simulink model "ppo_position_attitude4drone"  (R2025a)
settings: Solver=ode4  StartTime=0.0  StopTime=50  FixedStep=0.01  RelTol=1e-3
values from neighbouring files (symbols this model uses):
  control_noise = 0.045    [PPO_simulation.mat]    (also in TEST_POS_ATT_PPO.m)
  p_IC = IC(10)    [TEST_POS_ATT_PPO.m]
  phi_IC = IC(7)    [TEST_POS_ATT_PPO.m]
  psi_IC = IC(9)    [TEST_POS_ATT_PPO.m]
  q_IC = IC(11)    [TEST_POS_ATT_PPO.m]
  r_IC = IC(12)    [TEST_POS_ATT_PPO.m]
  state_noise = 0.045    [PPO_simulation.mat]    (also in TEST_POS_ATT_PPO.m)
  theta_IC = IC(8)    [TEST_POS_ATT_PPO.m]
  Ts_Sim = 0.01    [PPO_simulation.mat]    (also in TEST_POS_ATT_PPO.m)
  u_IC = IC(4)    [TEST_POS_ATT_PPO.m]
  v_IC = IC(5)    [TEST_POS_ATT_PPO.m]
  w_IC = IC(6)    [TEST_POS_ATT_PPO.m]
  x_IC = IC(1)    [TEST_POS_ATT_PPO.m]
  y_IC = IC(2)    [TEST_POS_ATT_PPO.m]
  z_IC = IC(3)    [TEST_POS_ATT_PPO.m]
undefined symbols (not defined in the file or in its folder): p_IC2, p_IC3, p_IC4, phi_IC2, phi_IC3, psi_IC2, psi_IC3, q_IC2, q_IC3, r_IC2, r_IC3, saturation_logic, theta_IC2, theta_IC3, u_IC2, u_IC3, v_IC2, v_IC3, w_IC2, w_IC3, wind_logic, x_IC2, x_IC3, y_IC2, y_IC3, z_IC2, z_IC3
libraries: rllib x8
(part 2 of 2)

== matlab function ppo_position_attitude4drone/drone2/Drone_Dynamic1/MATLAB Function5 ==
  data: X input; Wxyz input; X output; Ts_Sim input; wind_logic input
function X = wind_f_m( X,Wxyz, Ts_Sim,  wind_logic)

    Cd = [.8; 0.8;1.2]; % Drag coefficient
    L = 0.2; % Half arm length (m)
    h = 0.05;
    A = [L*2*h, L*2*h, 2*L*L]; % Approximate frontal areas [x, y, z] in m^2
    r = [ L,  L, -L, -L;   % X positions of motors
          L, -L, -L,  L;   % Y positions of motors
          0,  0,  0,  0 ]; % Z positions (motors at same height)
    rho = 1.225; % Air density (kg/m^3)

    Ix = 0.3; Iy = 0.4; Iz = 0.5; m = 1;
    if wind_logic ==1
        R = eul2rotm_zyx( X(7), X(8), X(9) );
        Wxyz_body = R'*Wxyz;
        V_rel = X(4:6) - Wxyz_body;
        F_wind = -0.5 * rho * Cd .*diag(A) * (V_rel .* abs(V_rel)); % Compute wind forces
        
        F_wind_motors = repmat(F_wind, 1, 4) + 0.01*randn(3,4);
    
        M_wind_motors = cross(r, F_wind_motors, 1);
        M_wind = sum(M_wind_motors, 2);  
        
        accn_dist = F_wind/m;
        alpha_dist=    [M_wind(1)/Ix;
                        M_wind(2)/Iy;
                        M_wind(3)/Iz];
    
        X = X + Ts_Sim * [0;0;0;
                         accn_dist;
                         0;0;0;
                         alpha_dist];
    end
end

== matlab function ppo_position_attitude4drone/drone2/Drone_Dynamic1/MATLAB Function6 ==
  data: U input; out output; logic input
% saturation function
function out = saturate_controls(U, logic)

    if logic == 1

        ft = U(1);
        torques = [U(2); U(3); U(4)];
        m = 1;
        g = 9.81;
        L = 0.2;
        drag = 0.02; % (drag coef)
        max_Ft = 2*m*g;
        Tmin = 0;
        Tmax = max_Ft/4;
        max_torque = Tmax*L*2;
        max_yaw_torque = 0.7*max_torque;

        % saturate the torques to the max torque the drone can produce
        for p = 1:2 % sat the first 2
            if torques(p) > max_torque
                torques(p) = max_torque;
            elseif torques(p) < -max_torque
                torques(p) = -max_torque;
            end
        end
        if torques(3) > max_yaw_torque
            torques(3) = max_yaw_torque;
        elseif torques(3) < -max_yaw_torque
            torques(3) = -max_yaw_torque;
        end
        % solve for the thrust of each motor given those torques
        T1 = (ft - torques(1)/(2*L) - torques(2)/(2*L) + torques(3)/(4*drag)) / 4;
        T2 = (ft - torques(1)/(2*L) + torques(2)/(2*L) + torques(3)/(4*drag)) / 4;
        T3 = (ft + torques(1)/(2*L) - torques(2)/(2*L) - torques(3)/(4*drag)) / 4;
        T4 = (ft + torques(1)/(2*L) + torques(2)/(2*L) - torques(3)/(4*drag)) / 4;
        each_motor_thrust = [T1;T2;T3;T4];

        % saturate each motor thrust to its bounded values
        for j = 1:4
            if each_motor_thrust(j) > Tmax
                each_motor_thrust(j) = Tmax;
            elseif each_motor_thrust(j) < Tmin
                each_motor_thrust(j) = Tmin;
            end
        end

        ft = sum(each_motor_thrust);

        if ft>max_Ft
            ft = max_Ft;
        elseif ft<0
            ft = 0;
        end

        out = [ft; torques];

    else
    
        out = U;
    
    end


end

== matlab function ppo_position_attitude4drone/drone2/Drone_Dynamic1/linear transfomation ==
  data: p input; q input; r input; phi_dot output; phi input; theta input; theta_dot output; psi_dot output
function [phi_dot, theta_dot, psi_dot] = fcn(p,q,r, phi,theta)

    phi_dot   = p + (q*sin(phi)*tan(theta)) + (r*cos(phi)*tan(theta));
    theta_dot = (q*cos(phi)) - (r*sin(phi));
    psi_dot   = (q*sin(phi)/cos(theta)) + (r*cos(phi)/cos(theta));

end



    % if theta == deg2rad(90) || theta == deg2rad(-90)
    %    theta = sign(theta)*deg2rad(89.9); 
    % end

% 89.9 value is fixed. 
% if change to 89.99, phi_dot and psi_dot value will explode.

== matlab function ppo_position_attitude4drone/leader drone/PPO_position_controller/Reward Function ==
  data: err input; u input; reward output
function reward  = fcn(err, u)

    % reward = -0.1 * (err.' * Q_pos * err + u.' * R_pos * u);
    err1 = err(1); % x
    err2 = err(2); % x_dot
    err3 = err(3);
    err4 = err(4);
    err5 = err(5);
    err6 = err(6);

    ux = u(1);
    uy = u(2);
    uz = u(3);

    reward = -0.05*(1*abs(err1) + 0.1*abs(err2) + 1*abs(err3) + 0.1*abs(err4) + ...
                    1*abs(err5) + 0.1*abs(err6) + 0.1*abs(ux) + 0.1*abs(uy) + 0.1*abs(uz));

end

== matlab function ppo_position_attitude4drone/drone2/PPO_attitude_controller/MATLAB Function1 ==
  data: err input; reward output; u input
function reward = fcn(err,u)
    err1 = err(1); % phi
    err2 = err(2); % phi_dot
    err3 = err(3);
    err4 = err(4);
    err5 = err(5);
    err6 = err(6);

    ux = u(1);
    uy = u(2);
    uz = u(3);

    reward = -1*(1*abs(err1) + 0.1*abs(err2) + 1*abs(err3) + 0.1*abs(err4) + ...
                    1*abs(err5) + 0.1*abs(err6) + 0.1*abs(ux) + 0.1*abs(uy) + 0.01*abs(uz));

end

== matlab function ppo_position_attitude4drone/drone2/PPO_position_controller/Reward Function ==
  data: err input; u input; reward output
function reward  = fcn(err, u)

    % reward = -0.1 * (err.' * Q_pos * err + u.' * R_pos * u);
    err1 = err(1); % x
    err2 = err(2); % x_dot
    err3 = err(3);
    err4 = err(4);
    err5 = err(5);
    err6 = err(6);

    ux = u(1);
    uy = u(2);
    uz = u(3);

    reward = -0.05*(1*abs(err1) + 0.1*abs(err2) + 1*abs(err3) + 0.1*abs(err4) + ...
                    1*abs(err5) + 0.1*abs(err6) + 0.1*abs(ux) + 0.1*abs(uy) + 0.1*abs(uz));

end

== matlab function ppo_position_attitude4drone/drone2/System_Solver ==
  data: phi_desired output; theta_desired output; psi_desired output; u_x input; Ft_desired output; u_y input; u_z input; t input
function [phi_desired, theta_desired, psi_desired, Ft_desired] = fcn(u_x, u_y, u_z, t)
    
    m = 1;
    psi_desired = 0.09;
    u_z = 9.81-u_z;
    Ft_desired = m * sqrt(u_x^2 + u_y^2 + u_z^2);
    phi_desired = asin((u_y*m)/Ft_desired);
    theta_desired = asin((-u_x*m) / (Ft_desired*cos(phi_desired)));

    %% the method below should work identically, use either 
    % a = sin(psi_desired); %sin(0) = 0
    % b = cos(psi_desired); %cos(0) = 1
    % A = u_x/u_z;
    % B = u_y/u_z;
    % C = (a*A - b*B) / ( (a^2) + (b^2));
    % phi_desired = atan((B + b*C) / a);
    % theta_desired = atan(C * cos(phi_desired));
    %%
    phi_desired = phi_desired *(1-exp(-2*t));
    theta_desired = theta_desired * (1-exp(-2*t));
    if phi_desired > pi/6
        phi_desired = pi/6;
    elseif phi_desired < -pi/6
        phi_desired = -pi/6;
    end
    %%
    if theta_desired > pi/6
        theta_desired = pi/6;
    elseif theta_desired < -pi/6
        theta_desired = -pi/6;
    end
    % Ft_desired = (m / (cos(theta_desired) * cos(phi_desired))) * (-u_z);
end

== matlab function ppo_position_attitude4drone/drone3/Drone_Dynamic1/MATLAB Function ==
  data: tau_x input; tau_y input; tau_z input; phi_d_dot output; theta_d_dot output; psi_d_dot output; phi_dot input; theta_dot input; psi_dot input
function [phi_d_dot, theta_d_dot, psi_d_dot] = fcn(tau_x, tau_y, tau_z, phi_dot, theta_dot, psi_dot)
    I_x = 0.3; I_y = 0.4; I_z = 0.5;
    phi_d_dot = (((I_y - I_z)/I_x) * theta_dot * psi_dot) + (tau_x/I_x);
    theta_d_dot = (((I_z - I_x)/I_y) * phi_dot * psi_dot) + (tau_y/I_y);
    psi_d_dot = (((I_x - I_y)/I_z) * phi_dot * psi_dot) + (tau_z/I_z);
end

== matlab function ppo_position_attitude4drone/drone3/Drone_Dynamic1/MATLAB Function1 ==
  data: phi input; x_d_dot output; theta input; psi input; F_t input; y_d_dot output; z_d_dot output
function [x_d_dot, y_d_dot, z_d_dot] = fcn(phi, theta, psi, F_t)
    m = 1; %1kg
    g = 9.81;
    x_d_dot= -(F_t/m) * (sin(phi)*sin(psi) + cos(phi)*cos(psi)*sin(theta));
    y_d_dot= -(F_t/m) * (cos(phi)*sin(psi)*sin(theta) - cos(psi)*sin(phi));
    z_d_dot= g-(F_t/m) * (cos(phi) * cos(theta));
end

== matlab function ppo_position_attitude4drone/drone3/Drone_Dynamic1/MATLAB Function3 ==
  settings: updateMethod=DISCRETE
  data: state_vector input; noisy_vector output; noise_percent input
function noisy_vector = add_state_noise(state_vector,noise_percent)

    sensor_uncert = [0.02, 0.02, 0.05, 0.05, 0.05, 0.05, 0.15, 0.15, 0.5, 0.005, 0.005, 0.005]';
  
    noise = (noise_percent) * sensor_uncert .* randn(size(state_vector)); % 0.01 usually add noise_percent 1 2 3 4 5
    noisy_vector = state_vector + noise;

end

== matlab function ppo_position_attitude4drone/drone3/Drone_Dynamic1/MATLAB Function4 ==
  settings: updateMethod=DISCRETE
  data: control_vector input; noisy_vector output; noise_percent input
function noisy_vector = add_control_noise(control_vector, noise_percent)

    L = 0.2;
    % drag = 0.02; % (drag coef)
    max_Ft = 2*9.81;
    Tmax = max_Ft/4;
    Max_torque = Tmax*L*2;
    actuator_uncert = [0.1*max_Ft, 0.01*Max_torque, 0.01*Max_torque, 0.02*Max_torque]';
    
    noise = (noise_percent) * actuator_uncert .* randn(size(control_vector)); % noise_percent 1 2 3 4 5
    noisy_vector = control_vector + noise;
    
end

== matlab function ppo_position_attitude4drone/drone3/Drone_Dynamic1/MATLAB Function5 ==
  data: X input; Wxyz input; X output; Ts_Sim input; wind_logic input
function X = wind_f_m( X,Wxyz, Ts_Sim,  wind_logic)

    Cd = [.8; 0.8;1.2]; % Drag coefficient
    L = 0.2; % Half arm length (m)
    h = 0.05;
    A = [L*2*h, L*2*h, 2*L*L]; % Approximate frontal areas [x, y, z] in m^2
    r = [ L,  L, -L, -L;   % X positions of motors
          L, -L, -L,  L;   % Y positions of motors
          0,  0,  0,  0 ]; % Z positions (motors at same height)
    rho = 1.225; % Air density (kg/m^3)

    Ix = 0.3; Iy = 0.4; Iz = 0.5; m = 1;
    if wind_logic ==1
        R = eul2rotm_zyx( X(7), X(8), X(9) );
        Wxyz_body = R'*Wxyz;
        V_rel = X(4:6) - Wxyz_body;
        F_wind = -0.5 * rho * Cd .*diag(A) * (V_rel .* abs(V_rel)); % Compute wind forces
        
        F_wind_motors = repmat(F_wind, 1, 4) + 0.01*randn(3,4);
    
        M_wind_motors = cross(r, F_wind_motors, 1);
        M_wind = sum(M_wind_motors, 2);  
        
        accn_dist = F_wind/m;
        alpha_dist=    [M_wind(1)/Ix;
                        M_wind(2)/Iy;
                        M_wind(3)/Iz];
    
        X = X + Ts_Sim * [0;0;0;
                         accn_dist;
                         0;0;0;
                         alpha_dist];
    end
end

== matlab function ppo_position_attitude4drone/leader drone/System_Solver ==
  data: phi_desired output; theta_desired output; psi_desired output; u_x input; Ft_desired output; u_y input; u_z input; t input
function [phi_desired, theta_desired, psi_desired, Ft_desired] = fcn(u_x, u_y, u_z, t)
    
    m = 1;
    psi_desired = 0.09;
    u_z = 9.81-u_z;
    Ft_desired = m * sqrt(u_x^2 + u_y^2 + u_z^2);
    phi_desired = asin((u_y*m)/Ft_desired);
    theta_desired = asin((-u_x*m) / (Ft_desired*cos(phi_desired)));

    %% the method below should work identically, use either 
    % a = sin(psi_desired); %sin(0) = 0
    % b = cos(psi_desired); %cos(0) = 1
    % A = u_x/u_z;
    % B = u_y/u_z;
    % C = (a*A - b*B) / ( (a^2) + (b^2));
    % phi_desired = atan((B + b*C) / a);
    % theta_desired = atan(C * cos(phi_desired));
    %%
    phi_desired = phi_desired *(1-exp(-2*t));
    theta_desired = theta_desired * (1-exp(-2*t));
    if phi_desired > pi/6
        phi_desired = pi/6;
    elseif phi_desired < -pi/6
        phi_desired = -pi/6;
    end
    %%
    if theta_desired > pi/6
        theta_desired = pi/6;
    elseif theta_desired < -pi/6
        theta_desired = -pi/6;
    end
    % Ft_desired = (m / (cos(theta_desired) * cos(phi_desired))) * (-u_z);
end

== matlab function ppo_position_attitude4drone/drone3/Drone_Dynamic1/MATLAB Function6 ==
  data: U input; out output; logic input
% saturation function
function out = saturate_controls(U, logic)

    if logic == 1

        ft = U(1);
        torques = [U(2); U(3); U(4)];
        m = 1;
        g = 9.81;
        L = 0.2;
        drag = 0.02; % (drag coef)
        max_Ft = 2*m*g;
        Tmin = 0;
        Tmax = max_Ft/4;
        max_torque = Tmax*L*2;
        max_yaw_torque = 0.7*max_torque;

        % saturate the torques to the max torque the drone can produce
        for p = 1:2 % sat the first 2
            if torques(p) > max_torque
                torques(p) = max_torque;
            elseif torques(p) < -max_torque
                torques(p) = -max_torque;
            end
        end
        if torques(3) > max_yaw_torque
            torques(3) = max_yaw_torque;
        elseif torques(3) < -max_yaw_torque
            torques(3) = -max_yaw_torque;
        end
        % solve for the thrust of each motor given those torques
        T1 = (ft - torques(1)/(2*L) - torques(2)/(2*L) + torques(3)/(4*drag)) / 4;
        T2 = (ft - torques(1)/(2*L) + torques(2)/(2*L) + torques(3)/(4*drag)) / 4;
        T3 = (ft + torques(1)/(2*L) - torques(2)/(2*L) - torques(3)/(4*drag)) / 4;
        T4 = (ft + torques(1)/(2*L) + torques(2)/(2*L) - torques(3)/(4*drag)) / 4;
        each_motor_thrust = [T1;T2;T3;T4];

        % saturate each motor thrust to its bounded values
        for j = 1:4
            if each_motor_thrust(j) > Tmax
                each_motor_thrust(j) = Tmax;
            elseif each_motor_thrust(j) < Tmin
                each_motor_thrust(j) = Tmin;
            end
        end

        ft = sum(each_motor_thrust);

        if ft>max_Ft
            ft = max_Ft;
        elseif ft<0
            ft = 0;
        end

        out = [ft; torques];

    else
    
        out = U;
    
    end


end

== matlab function ppo_position_attitude4drone/drone3/Drone_Dynamic1/linear transfomation ==
  data: p input; q input; r input; phi_dot output; phi input; theta input; theta_dot output; psi_dot output
function [phi_dot, theta_dot, psi_dot] = fcn(p,q,r, phi,theta)

    phi_dot   = p + (q*sin(phi)*tan(theta)) + (r*cos(phi)*tan(theta));
    theta_dot = (q*cos(phi)) - (r*sin(phi));
    psi_dot   = (q*sin(phi)/cos(theta)) + (r*cos(phi)/cos(theta));

end



    % if theta == deg2rad(90) || theta == deg2rad(-90)
    %    theta = sign(theta)*deg2rad(89.9); 
    % end

% 89.9 value is fixed. 
% if change to 89.99, phi_dot and psi_dot value will explode.

== matlab function ppo_position_attitude4drone/drone3/PPO_attitude_controller/MATLAB Function1 ==
  data: err input; reward output; u input
function reward = fcn(err,u)
    err1 = err(1); % phi
    err2 = err(2); % phi_dot
    err3 = err(3);
    err4 = err(4);
    err5 = err(5);
    err6 = err(6);

    ux = u(1);
    uy = u(2);
    uz = u(3);

    reward = -1*(1*abs(err1) + 0.1*abs(err2) + 1*abs(err3) + 0.1*abs(err4) + ...
                    1*abs(err5) + 0.1*abs(err6) + 0.1*abs(ux) + 0.1*abs(uy) + 0.01*abs(uz));

end

== matlab function ppo_position_attitude4drone/drone3/PPO_position_controller/Reward Function ==
  data: err input; u input; reward output
function reward  = fcn(err, u)

    % reward = -0.1 * (err.' * Q_pos * err + u.' * R_pos * u);
    err1 = err(1); % x
    err2 = err(2); % x_dot
    err3 = err(3);
    err4 = err(4);
    err5 = err(5);
    err6 = err(6);

    ux = u(1);
    uy = u(2);
    uz = u(3);

    reward = -0.05*(1*abs(err1) + 0.1*abs(err2) + 1*abs(err3) + 0.1*abs(err4) + ...
                    1*abs(err5) + 0.1*abs(err6) + 0.1*abs(ux) + 0.1*abs(uy) + 0.1*abs(uz));

end

== matlab function ppo_position_attitude4drone/drone3/System_Solver ==
  data: phi_desired output; theta_desired output; psi_desired output; u_x input; Ft_desired output; u_y input; u_z input; t input
function [phi_desired, theta_desired, psi_desired, Ft_desired] = fcn(u_x, u_y, u_z, t)
    
    m = 1;
    psi_desired = 0.09;
    u_z = 9.81-u_z;
    Ft_desired = m * sqrt(u_x^2 + u_y^2 + u_z^2);
    phi_desired = asin((u_y*m)/Ft_desired);
    theta_desired = asin((-u_x*m) / (Ft_desired*cos(phi_desired)));

    %% the method below should work identically, use either 
    % a = sin(psi_desired); %sin(0) = 0
    % b = cos(psi_desired); %cos(0) = 1
    % A = u_x/u_z;
    % B = u_y/u_z;
    % C = (a*A - b*B) / ( (a^2) + (b^2));
    % phi_desired = atan((B + b*C) / a);
    % theta_desired = atan(C * cos(phi_desired));
    %%
    phi_desired = phi_desired *(1-exp(-2*t));
    theta_desired = theta_desired * (1-exp(-2*t));
    if phi_desired > pi/6
        phi_desired = pi/6;
    elseif phi_desired < -pi/6
        phi_desired = -pi/6;
    end
    %%
    if theta_desired > pi/6
        theta_desired = pi/6;
    elseif theta_desired < -pi/6
        theta_desired = -pi/6;
    end
    % Ft_desired = (m / (cos(theta_desired) * cos(phi_desired))) * (-u_z);
end

== matlab function ppo_position_attitude4drone/drone4/Drone_Dynamic1/MATLAB Function1 ==
  data: phi input; x_d_dot output; theta input; psi input; F_t input; y_d_dot output; z_d_dot output
function [x_d_dot, y_d_dot, z_d_dot] = fcn(phi, theta, psi, F_t)
    m = 1; %1kg
    g = 9.81;
    x_d_dot= -(F_t/m) * (sin(phi)*sin(psi) + cos(phi)*cos(psi)*sin(theta));
    y_d_dot= -(F_t/m) * (cos(phi)*sin(psi)*sin(theta) - cos(psi)*sin(phi));
    z_d_dot= g-(F_t/m) * (cos(phi) * cos(theta));
end

== matlab function ppo_position_attitude4drone/drone4/Drone_Dynamic1/MATLAB Function3 ==
  settings: updateMethod=DISCRETE
  data: state_vector input; noisy_vector output; noise_percent input
function noisy_vector = add_state_noise(state_vector,noise_percent)

    sensor_uncert = [0.02, 0.02, 0.05, 0.05, 0.05, 0.05, 0.15, 0.15, 0.5, 0.005, 0.005, 0.005]';
  
    noise = (noise_percent) * sensor_uncert .* randn(size(state_vector)); % 0.01 usually add noise_percent 1 2 3 4 5
    noisy_vector = state_vector + noise;

end

== matlab function ppo_position_attitude4drone/drone4/Drone_Dynamic1/MATLAB Function4 ==
  settings: updateMethod=DISCRETE
  data: control_vector input; noisy_vector output; noise_percent input
function noisy_vector = add_control_noise(control_vector, noise_percent)

    L = 0.2;
    % drag = 0.02; % (drag coef)
    max_Ft = 2*9.81;
    Tmax = max_Ft/4;
    Max_torque = Tmax*L*2;
    actuator_uncert = [0.1*max_Ft, 0.01*Max_torque, 0.01*Max_torque, 0.02*Max_torque]';
    
    noise = (noise_percent) * actuator_uncert .* randn(size(control_vector)); % noise_percent 1 2 3 4 5
    noisy_vector = control_vector + noise;
    
end

== matlab function ppo_position_attitude4drone/drone4/Drone_Dynamic1/MATLAB Function5 ==
  data: X input; Wxyz input; X output; Ts_Sim input; wind_logic input
function X = wind_f_m( X,Wxyz, Ts_Sim,  wind_logic)

    Cd = [.8; 0.8;1.2]; % Drag coefficient
    L = 0.2; % Half arm length (m)
    h = 0.05;
    A = [L*2*h, L*2*h, 2*L*L]; % Approximate frontal areas [x, y, z] in m^2
    r = [ L,  L, -L, -L;   % X positions of motors
          L, -L, -L,  L;   % Y positions of motors
          0,  0,  0,  0 ]; % Z positions (motors at same height)
    rho = 1.225; % Air density (kg/m^3)

    Ix = 0.3; Iy = 0.4; Iz = 0.5; m = 1;
    if wind_logic ==1
        R = eul2rotm_zyx( X(7), X(8), X(9) );
        Wxyz_body = R'*Wxyz;
        V_rel = X(4:6) - Wxyz_body;
        F_wind = -0.5 * rho * Cd .*diag(A) * (V_rel .* abs(V_rel)); % Compute wind forces
        
        F_wind_motors = repmat(F_wind, 1, 4) + 0.01*randn(3,4);
    
        M_wind_motors = cross(r, F_wind_motors, 1);
        M_wind = sum(M_wind_motors, 2);  
        
        accn_dist = F_wind/m;
        alpha_dist=    [M_wind(1)/Ix;
                        M_wind(2)/Iy;
                        M_wind(3)/Iz];
    
        X = X + Ts_Sim * [0;0;0;
                         accn_dist;
                         0;0;0;
                         alpha_dist];
    end
end

== matlab function ppo_position_attitude4drone/drone4/Drone_Dynamic1/MATLAB Function6 ==
  data: U input; out output; logic input
% saturation function
function out = saturate_controls(U, logic)

    if logic == 1

        ft = U(1);
        torques = [U(2); U(3); U(4)];
        m = 1;
        g = 9.81;
        L = 0.2;
        drag = 0.02; % (drag coef)
        max_Ft = 2*m*g;
        Tmin = 0;
        Tmax = max_Ft/4;
        max_torque = Tmax*L*2;
        max_yaw_torque = 0.7*max_torque;

        % saturate the torques to the max torque the drone can produce
        for p = 1:2 % sat the first 2
            if torques(p) > max_torque
                torques(p) = max_torque;
            elseif torques(p) < -max_torque
                torques(p) = -max_torque;
            end
        end
        if torques(3) > max_yaw_torque
            torques(3) = max_yaw_torque;
        elseif torques(3) < -max_yaw_torque
            torques(3) = -max_yaw_torque;
        end
        % solve for the thrust of each motor given those torques
        T1 = (ft - torques(1)/(2*L) - torques(2)/(2*L) + torques(3)/(4*drag)) / 4;
        T2 = (ft - torques(1)/(2*L) + torques(2)/(2*L) + torques(3)/(4*drag)) / 4;
        T3 = (ft + torques(1)/(2*L) - torques(2)/(2*L) - torques(3)/(4*drag)) / 4;
        T4 = (ft + torques(1)/(2*L) + torques(2)/(2*L) - torques(3)/(4*drag)) / 4;
        each_motor_thrust = [T1;T2;T3;T4];

        % saturate each motor thrust to its bounded values
        for j = 1:4
            if each_motor_thrust(j) > Tmax
                each_motor_thrust(j) = Tmax;
            elseif each_motor_thrust(j) < Tmin
                each_motor_thrust(j) = Tmin;
            end
        end

        ft = sum(each_motor_thrust);

        if ft>max_Ft
            ft = max_Ft;
        elseif ft<0
            ft = 0;
        end

        out = [ft; torques];

    else
    
        out = U;
    
    end


end

== matlab function ppo_position_attitude4drone/drone4/Drone_Dynamic1/linear transfomation ==
  data: p input; q input; r input; phi_dot output; phi input; theta input; theta_dot output; psi_dot output
function [phi_dot, theta_dot, psi_dot] = fcn(p,q,r, phi,theta)

    phi_dot   = p + (q*sin(phi)*tan(theta)) + (r*cos(phi)*tan(theta));
    theta_dot = (q*cos(phi)) - (r*sin(phi));
    psi_dot   = (q*sin(phi)/cos(theta)) + (r*cos(phi)/cos(theta));

end



    % if theta == deg2rad(90) || theta == deg2rad(-90)
    %    theta = sign(theta)*deg2rad(89.9); 
    % end

% 89.9 value is fixed. 
% if change to 89.99, phi_dot and psi_dot value will explode.

== matlab function ppo_position_attitude4drone/drone4/PPO_attitude_controller/MATLAB Function1 ==
  data: err input; reward output; u input
function reward = fcn(err,u)
    err1 = err(1); % phi
    err2 = err(2); % phi_dot
    err3 = err(3);
    err4 = err(4);
    err5 = err(5);
    err6 = err(6);

    ux = u(1);
    uy = u(2);
    uz = u(3);

    reward = -1*(1*abs(err1) + 0.1*abs(err2) + 1*abs(err3) + 0.1*abs(err4) + ...
                    1*abs(err5) + 0.1*abs(err6) + 0.1*abs(ux) + 0.1*abs(uy) + 0.01*abs(uz));

end

== matlab function ppo_position_attitude4drone/drone4/PPO_position_controller/Reward Function ==
  data: err input; u input; reward output
function reward  = fcn(err, u)

    % reward = -0.1 * (err.' * Q_pos * err + u.' * R_pos * u);
    err1 = err(1); % x
    err2 = err(2); % x_dot
    err3 = err(3);
    err4 = err(4);
    err5 = err(5);
    err6 = err(6);

    ux = u(1);
    uy = u(2);
    uz = u(3);

    reward = -0.05*(1*abs(err1) + 0.1*abs(err2) + 1*abs(err3) + 0.1*abs(err4) + ...
                    1*abs(err5) + 0.1*abs(err6) + 0.1*abs(ux) + 0.1*abs(uy) + 0.1*abs(uz));

end

== matlab function ppo_position_attitude4drone/drone4/System_Solver ==
  data: phi_desired output; theta_desired output; psi_desired output; u_x input; Ft_desired output; u_y input; u_z input; t input
function [phi_desired, theta_desired, psi_desired, Ft_desired] = fcn(u_x, u_y, u_z, t)
    
    m = 1;
    psi_desired = 0.09;
    u_z = 9.81-u_z;
    Ft_desired = m * sqrt(u_x^2 + u_y^2 + u_z^2);
    phi_desired = asin((u_y*m)/Ft_desired);
    theta_desired = asin((-u_x*m) / (Ft_desired*cos(phi_desired)));

    %% the method below should work identically, use either 
    % a = sin(psi_desired); %sin(0) = 0
    % b = cos(psi_desired); %cos(0) = 1
    % A = u_x/u_z;
    % B = u_y/u_z;
    % C = (a*A - b*B) / ( (a^2) + (b^2));
    % phi_desired = atan((B + b*C) / a);
    % theta_desired = atan(C * cos(phi_desired));
    %%
    phi_desired = phi_desired *(1-exp(-2*t));
    theta_desired = theta_desired * (1-exp(-2*t));
    if phi_desired > pi/6
        phi_desired = pi/6;
    elseif phi_desired < -pi/6
        phi_desired = -pi/6;
    end
    %%
    if theta_desired > pi/6
        theta_desired = pi/6;
    elseif theta_desired < -pi/6
        theta_desired = -pi/6;
    end
    % Ft_desired = (m / (cos(theta_desired) * cos(phi_desired))) * (-u_z);
end

== matlab function ppo_position_attitude4drone/leader drone/Drone_Dynamic1/MATLAB Function5 ==
  data: X input; Wxyz input; X output; Ts_Sim input; wind_logic input
function X = wind_f_m( X,Wxyz, Ts_Sim,  wind_logic)

    Cd = [.8; 0.8;1.2]; % Drag coefficient
    L = 0.2; % Half arm length (m)
    h = 0.05;
    A = [L*2*h, L*2*h, 2*L*L]; % Approximate frontal areas [x, y, z] in m^2
    r = [ L,  L, -L, -L;   % X positions of motors
          L, -L, -L,  L;   % Y positions of motors
          0,  0,  0,  0 ]; % Z positions (motors at same height)
    rho = 1.225; % Air density (kg/m^3)

    Ix = 0.3; Iy = 0.4; Iz = 0.5; m = 1;
    if wind_logic ==1
        R = eul2rotm_zyx( X(7), X(8), X(9) );
        Wxyz_body = R'*Wxyz;
        V_rel = X(4:6) - Wxyz_body;
        F_wind = -0.5 * rho * Cd .*diag(A) * (V_rel .* abs(V_rel)); % Compute wind forces
        
        F_wind_motors = repmat(F_wind, 1, 4) + 0.01*randn(3,4);
    
        M_wind_motors = cross(r, F_wind_motors, 1);
        M_wind = sum(M_wind_motors, 2);  
        
        accn_dist = F_wind/m;
        alpha_dist=    [M_wind(1)/Ix;
                        M_wind(2)/Iy;
                        M_wind(3)/Iz];
    
        X = X + Ts_Sim * [0;0;0;
                         accn_dist;
                         0;0;0;
                         alpha_dist];
    end
end

== matlab function ppo_position_attitude4drone/Ref Mixer ==
  data: t input; leader input; drone2 input; drone3 input; drone4 input; ref2 output; ref3 output; ref4 output
function [ref2, ref3, ref4] = fcn(t, leader, drone2, drone3, drone4)
ref2 = zeros(6,1);
ref3 = zeros(6,1);
ref4 = zeros(6,1);
N = 5000;
N1 = floor(N/3);
N2 = floor(2*N/3);

comm = 0;
offsets = zeros(3, 4);
offsets(:,1) = [ 0;  0; 0];
offsets(:,2) = [-1;  0; 0];
offsets(:,3) = [-1; -1; 0];
offsets(:,4) = [-1;  1; 0];
X1 = zeros(6,1);
X2 = zeros(6,1);
X3 = zeros(6,1);
X4 = zeros(6,1);

% eddie uses a weird vector format
% go from x xd y yd z zd => x y z xd yd zd (1,3,5,2,4,6)
X1 = [leader(1); leader(3); leader(5);leader(2);leader(4);leader(6)];

X2 = [drone2(1);drone2(3);drone2(5);drone2(2);drone2(4);drone2(6)];
X3 = [drone3(1);drone3(3);drone3(5);drone3(2);drone3(4);drone3(6)];
X4 = [drone4(1);drone4(3);drone4(5);drone4(2);drone4(4);drone4(6)];

    if comm == 0
        ref2 = [X1(1:3) + offsets(:,2); X1(4:6)];
        ref3 = [X1(1:3) + offsets(:,3); X1(4:6)];
        ref4 = [X1(1:3) + offsets(:,4); X1(4:6)];
    elseif comm == 1
        if t <= (N1/2)*.01
            ref2 = [X1(1:3) + offsets(:,2); X1(4:6)];
            ref3 = [X1(1:3) + offsets(:,3); X1(4:6)];
            ref4 = [X1(1:3) + offsets(:,4); X1(4:6)];
        elseif t <= N1*.01 && t > (N1/2)*.01
            ref2 = [X3(1:3) + (offsets(:,2) - offsets(:,3));   X3(4:6)]; % 2 only sees 3
            ref3 = [X1(1:3) + offsets(:,3);                    X1(4:6)]; % 2 only sees leader
            ref4 = [X2(1:3) + (offsets(:,4) - offsets(:,2));   X2(4:6)]; % 4 only sees 2
        elseif t <= N2*.01 && t > N1*.01
            ref2 = [X1(1:3) + offsets(:,2);                    X1(4:6)]; % 2 only sees leader
            ref3 = [X2(1:3) + (offsets(:,3) - offsets(:,2));   X2(4:6)]; % 3 only sees 2
            ref4 = [X3(1:3) + (offsets(:,4) - offsets(:,3));   X3(4:6)]; % 4 only sees 3
        else
            ref2 = [X3(1:3) + (offsets(:,2) - offsets(:,3));   X3(4:6)]; % 2 only sees 3
            ref3 = [(X4(1:3) + (offsets(:,3)- offsets(:,4)));  X4(4:6)]; % 3 only sees 4
            ref4 = [X1(1:3) + offsets(:,4);                    X1(4:6)]; % 4 only sees leader
        end

    end
    % go from x y z xd yd zd => x xd y yd z zd (1,4,2,5,3,6)
    ref2 = [ref2(1); ref2(4); ref2(2); ref2(5); ref2(3); ref2(6)];
    ref3 = [ref3(1); ref3(4); ref3(2); ref3(5); ref3(3); ref3(6)];
    ref4 = [ref4(1); ref4(4); ref4(2); ref4(5); ref4(3); ref4(6)];
end

== matlab function ppo_position_attitude4drone/Reference Signals1/MATLAB Function ==
  data: t input; x_desir output; x_d_desir output; y_desir output; y_d_desir output; z_desir output; z_d_desir output
function [x_desir, x_d_desir, y_desir, y_d_desir,...
    z_desir, z_d_desir] = trajectory_generator(t)
% trajectory_generator generates desired position and velocity.
    
    % x_desir = 10 * sin(0.25*t);
    % x_d_desir = 2.5 * cos(0.25*t);
    % y_desir = 70 * (1-exp(-0.01*t)) * cos(0.2*t);
    % y_d_desir = 70*(0.01*exp(-0.01*t))*cos(0.2*t) - 14*(1-exp(-0.01*t))*sin(0.2*t);
    
    %% helix
    % x_desir = (1-exp(-0.01*t))*9.81*cos(0.2*t);
    % x_d_desir = 9.81 * (0.01 * exp(-0.01 * t) * cos(0.2 * t) - 0.2 * (1 - exp(-0.01 * t)) * sin(0.2 * t));
    % y_desir = (1-exp(-0.01*t))*9.81*sin(0.2*t);
    % y_d_desir =  9.81 * (0.2 * (1 - exp(-0.01*t)) * cos(0.2*t) + 0.01 * exp(-0.01*t) * sin(0.2*t));
    % z_desir = -0.1*t;
    % z_d_desir = -0.1;

    %% crown path 
    x_desir = 9.81*cos(0.2*t);
    x_d_desir = -1.962*sin(0.2*t);

    y_desir = 9.81*sin(0.2*t);
    y_d_desir =  1.962*cos(0.2*t);
    
    z_desir = -4*cos(1*t)-9.81;
    z_d_desir = 4*sin(t);

    % x_desir = 0;
    % x_d_desir = 0;
    % y_desir = 0;
    % y_d_desir =  0;
    % z_desir = -0.1*t;
    % z_d_desir = -0.1;
end

== matlab function ppo_position_attitude4drone/leader drone/Drone_Dynamic1/MATLAB Function3 ==
  settings: updateMethod=DISCRETE
  data: state_vector input; noisy_vector output; noise_percent input
function noisy_vector = add_state_noise(state_vector,noise_percent)

    sensor_uncert = [0.02, 0.02, 0.05, 0.05, 0.05, 0.05, 0.15, 0.15, 0.5, 0.005, 0.005, 0.005]';
  
    noise = (noise_percent) * sensor_uncert .* randn(size(state_vector)); % 0.01 usually add noise_percent 1 2 3 4 5
    noisy_vector = state_vector + noise;

end

== matlab function ppo_position_attitude4drone/leader drone/PPO_attitude_controller/MATLAB Function1 ==
  data: err input; reward output; u input
function reward = fcn(err,u)
    err1 = err(1); % phi
    err2 = err(2); % phi_dot
    err3 = err(3);
    err4 = err(4);
    err5 = err(5);
    err6 = err(6);

    ux = u(1);
    uy = u(2);
    uz = u(3);

    reward = -1*(1*abs(err1) + 0.1*abs(err2) + 1*abs(err3) + 0.1*abs(err4) + ...
                    1*abs(err5) + 0.1*abs(err6) + 0.1*abs(ux) + 0.1*abs(uy) + 0.01*abs(uz));

end

== matlab function ppo_position_attitude4drone/leader drone/Drone_Dynamic1/MATLAB Function ==
  data: tau_x input; tau_y input; tau_z input; phi_d_dot output; theta_d_dot output; psi_d_dot output; phi_dot input; theta_dot input; psi_dot input
function [phi_d_dot, theta_d_dot, psi_d_dot] = fcn(tau_x, tau_y, tau_z, phi_dot, theta_dot, psi_dot)
    I_x = 0.3; I_y = 0.4; I_z = 0.5;
    phi_d_dot = (((I_y - I_z)/I_x) * theta_dot * psi_dot) + (tau_x/I_x);
    theta_d_dot = (((I_z - I_x)/I_y) * phi_dot * psi_dot) + (tau_y/I_y);
    psi_d_dot = (((I_x - I_y)/I_z) * phi_dot * psi_dot) + (tau_z/I_z);
end

== matlab function ppo_position_attitude4drone/leader drone/Drone_Dynamic1/MATLAB Function1 ==
  data: phi input; x_d_dot output; theta input; psi input; F_t input; y_d_dot output; z_d_dot output
function [x_d_dot, y_d_dot, z_d_dot] = fcn(phi, theta, psi, F_t)
    m = 1; %1kg
    g = 9.81;
    x_d_dot= -(F_t/m) * (sin(phi)*sin(psi) + cos(phi)*cos(psi)*sin(theta));
    y_d_dot= -(F_t/m) * (cos(phi)*sin(psi)*sin(theta) - cos(psi)*sin(phi));
    z_d_dot= g-(F_t/m) * (cos(phi) * cos(theta));
end

== matlab function ppo_position_attitude4drone/drone4/Drone_Dynamic1/MATLAB Function ==
  data: tau_x input; tau_y input; tau_z input; phi_d_dot output; theta_d_dot output; psi_d_dot output; phi_dot input; theta_dot input; psi_dot input
function [phi_d_dot, theta_d_dot, psi_d_dot] = fcn(tau_x, tau_y, tau_z, phi_dot, theta_dot, psi_dot)
    I_x = 0.3; I_y = 0.4; I_z = 0.5;
    phi_d_dot = (((I_y - I_z)/I_x) * theta_dot * psi_dot) + (tau_x/I_x);
    theta_d_dot = (((I_z - I_x)/I_y) * phi_dot * psi_dot) + (tau_y/I_y);
    psi_d_dot = (((I_x - I_y)/I_z) * phi_dot * psi_dot) + (tau_z/I_z);
end
